simulink model "SpringMPCmimo"  (R2021a)
settings: Solver=FixedStepDiscrete  StartTime=0.0  StopTime=10.0  FixedStep=0.05  RelTol=1e-3
model workspace (MAT data in the model file):
  Asim = [-0.0455  -0.0273  -0.0273; -0.0273  -0.0455  -0.0273; -0.0273  -0.0273  -0.0455]
settings Model: Creator=iris  LastModifiedBy=iris
settings SolverCC: AlgebraicLoopSolver=TrustRegion

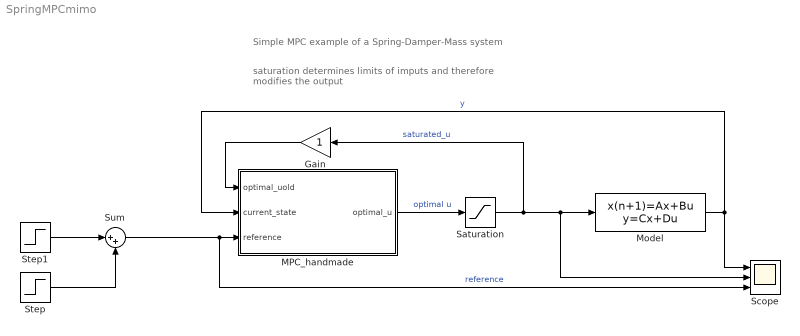
== system SpringMPCmimo ==
  note: saturation determines limits of imputs and therefore modifies the output
  note: Simple MPC example of a Spring-Damper-Mass system
  Gain : Gain
  MPC_handmade : MATLAB Function  TreatAsAtomicUnit=on
  Model : DiscreteStateSpace  A=|  B=|  C=eye(2)  D=zeros(2,1)  InitialCondition=[0 0]  SampleTime=-1
      A=|
      | [ 0.9988    0.0464;
      |    -0.0464    0.8596]
      B=|
      | [0.0012;
      |     0.0464]
  Saturation : Saturate  UpperLimit=100  LowerLimit=-5
  Scope : Scope  NumInputPorts=3
  Step : Step  Time=7  After=-2  SampleTime=0
  Step1 : Step  After=2  SampleTime=0
  Sum : Sum  Inputs=|++
  wires:
  Model/1 -> MPC_handmade/2(current_state), Scope/1  "y"
  MPC_handmade/1(optimal_u) -> Saturation/1  "optimal u"
  Step/1 -> Sum/2
  Step1/1 -> Sum/1
  Sum/1 -> Scope/3, MPC_handmade/3(reference)  "reference"
  Gain/1 -> MPC_handmade/1(optimal_uold)
  Saturation/1 -> Gain/1, Scope/2, Model/1  "saturated_u"

== matlab function SpringMPCmimo/MPC_handmade ==
  data: optimal_uold input; current_state input; reference input; optimal_u output
function optimal_u = MPCmimo_handmade(optimal_uold,current_state,reference)
% J = [8 -3 -3; -3 8 -3; -3 -3 8];
% F = 0.2*eye(3);
% Ap = -J\F;
% Bp = inv(J);
Cp = eye(2);
m = 1;
b = 3;
k = 1;
% Continuous matrices
Ac =[0 1; -k/m -b/m];
Bc =[0;1];
%%% Discrete after [Ad,Bd,Cd,Dd] = c2dm(Ap,Bp,Cp,Dp,Delta_t) with delta_t=
%%% 0.05
Ap = [ 0.9988    0.0464;
   -0.0464    0.8596];
Bp = [0.0012;
    0.0464];


% Dp = zeros(3);
Np = 10;
Nc = 4;
% persistent u_next
% if isempty(u_next)
%     u_next = 0;
% end
% MPC gains %%%%%%%%%%%%%%
[m1,n1] = size(Cp);
[n1,n_in] = size(Bp);
A_e = eye(n1+m1,n1+m1);
A_e(1:n1,1:n1) = Ap;
A_e(n1+1:n1+m1,1:n1) = Cp*Ap;
B_e = zeros(n1+m1,n_in);
B_e(1:n1,:) = Bp;
B_e(n1+1:n1+m1,:) = Cp*Bp;
C_e = zeros(m1,n1+m1);
C_e(:,n1+1:n1+m1) = eye(m1,m1);

n = n1+m1;
h = zeros(Np*m1,n1+m1);
F = zeros(Np*m1,size(C_e*A_e,2));
h(1:m1,:) = C_e;
F(1:m1,:) = C_e*A_e;
for kk = (m1+1):m1:Np*m1
    h(kk:kk+m1-1,:) = h(kk-m1:kk-1,:)*A_e;
    F(kk:kk+m1-1,:) = F(kk-m1:kk-1,:)*A_e;
end

v = h*B_e;
Phi = zeros(Np*m1,Nc*n_in);
Phi(:,1:n_in) = v;
for i=(n_in+1):n_in:Nc*n_in 
    Phi(:,i:i+n_in-1) = [zeros(i-m1,n_in);v(1:Np*m1-i+m1,:)]; %Toeplitz matrix
end
BarRs = ones(Np*m1,m1);
% for i = 1:Np*m1
%     BarRs(i,:)=reference;
% end
Phi_Phi = Phi'*Phi;
Phi_F = Phi'*F;
Phi_R = Phi_F(:,end-n_in+1:end);

%%%%%%%%%%%%%%%%%%%%%%%%%%%%%%%%%%
if isempty(optimal_uold)
    u_next = reference;
else
    u_next = optimal_uold;
end
 
BarR = 0.5*eye(size(Phi_Phi));
xm_next = Ap*current_state+Bp*u_next;
y_next = xm_next;
Delta_xm = xm_next-current_state;
x_next = [Delta_xm; xm_next];
optimal_DeltaU = (Phi_Phi+BarR)\(Phi_R*reference-Phi_F*x_next);
Ky = (Phi_Phi+BarR)\(Phi'*F(:,end))
Kmpc = (Phi_Phi+BarR)\(Phi'*F)
% eig(A_e-B_e*Kmpc)

u_next = u_next + optimal_DeltaU(1:n_in,:);
optimal_u = u_next;

%%%% Saturation of the optimal input is defined in the simulink model
